simulink subsystem "ROS2_Bball_MatPub"  (R2024b)
settings: Solver=VariableStepAuto  StartTime=0.0  StopTime=10.0  RelTol=1e-3
settings Model: Creator=macheson  LastModifiedBy=macheson

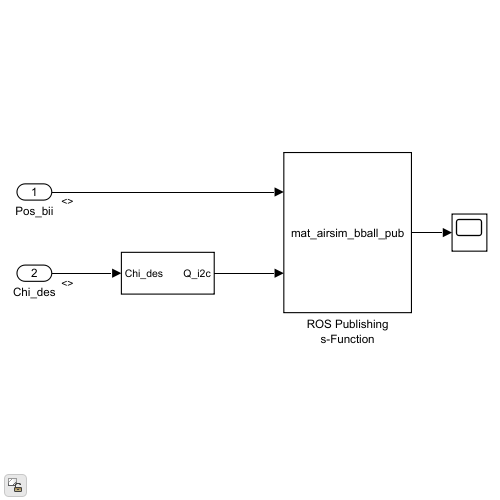
[thumbnail: Simulink's stored preview of the top-level diagram]
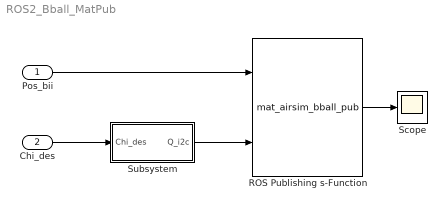
== system ROS2_Bball_MatPub ==
  Pos_bii : Inport
  Chi_des : Inport  Port=2
  ROS Publishing s-Function : S-Function  FunctionName=mat_airsim_bball_pub  SFunctionDeploymentMode=off  EnableBusSupport=off
  Scope : Scope
  Subsystem : Subsystem
  wires:
  ROS Publishing s-Function/1 -> Scope/1
  Pos_bii/1 -> ROS Publishing s-Function/1
  Chi_des/1 -> Subsystem/1(Chi_des)
  Subsystem/1(Q_i2c) -> ROS Publishing s-Function/2

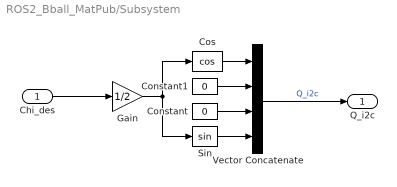
== system ROS2_Bball_MatPub/Subsystem ==
  Chi_des : Inport
  Constant : Constant  Value=0
  Constant1 : Constant  Value=0
  Cos : Trigonometry  Operator=cos
  Gain : Gain  Gain=1/2
  Sin : Trigonometry
  Vector Concatenate : Concatenate  NumInputs=4
  Q_i2c : Outport
  wires:
  Chi_des/1 -> Gain/1
  Constant1/1 -> Vector Concatenate/2
  Vector Concatenate/1 -> Q_i2c/1  "Q_i2c"
  Cos/1 -> Vector Concatenate/1
  Gain/1 -> Cos/1, Sin/1
  Sin/1 -> Vector Concatenate/4
  Constant/1 -> Vector Concatenate/3
